simulink model "Lab1bPartC1"  (R2023b)
settings: Solver=VariableStepAuto  StartTime=0.0  StopTime=150  RelTol=1e-3
settings Model: Creator=tanvi  LastModifiedBy=tanvi

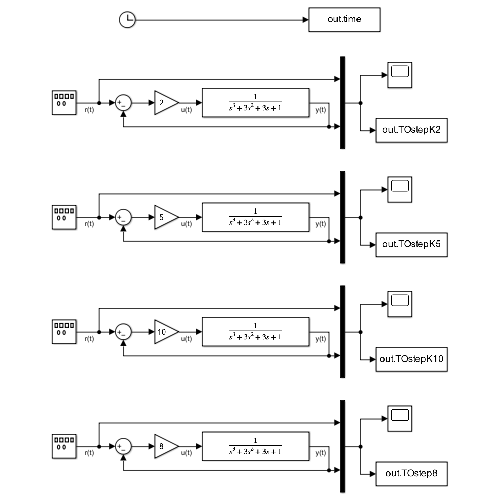
[thumbnail: Simulink's stored preview of the top-level diagram]
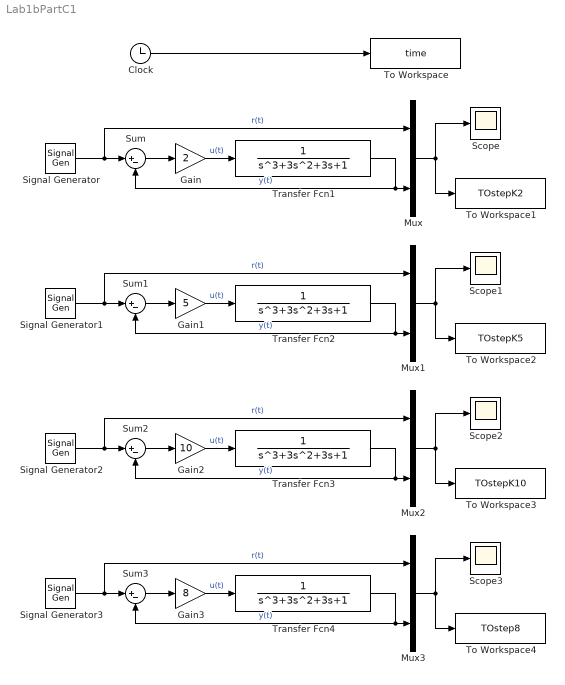
== system Lab1bPartC1 ==
  Clock : Clock
      settings: Decimation=100
  Gain : Gain  Gain=2
  Gain1 : Gain  Gain=5
  Gain2 : Gain  Gain=10
  Gain3 : Gain  Gain=8
  Mux{,1..3} (4 alike) : Mux  Inputs=2
  Scope{,1..3} (4 alike) : Scope
  Signal Generator{,1..3} (4 alike) : SignalGenerator  WaveForm=square  Frequency=0.01
  Sum{,1..3} (4 alike) : Sum  Inputs=|+-
  To Workspace : ToWorkspace  VariableName=time  SampleTime=-1
  To Workspace1 : ToWorkspace  VariableName=TOstepK2  SampleTime=-1
  To Workspace2 : ToWorkspace  VariableName=TOstepK5  SampleTime=-1
  To Workspace3 : ToWorkspace  VariableName=TOstepK10  SampleTime=-1
  To Workspace4 : ToWorkspace  VariableName=TOstep8  SampleTime=-1
  Transfer Fcn{1..4} (4 alike) : TransferFcn  Denominator=[1 3 3 1]
  wires:
  Mux/1 -> Scope/1, To Workspace1/1
  Clock/1 -> To Workspace/1
  Sum/1 -> Gain/1
  Gain/1 -> Transfer Fcn1/1  "u(t)"
  Transfer Fcn1/1 -> Sum/2, Mux/2  "y(t)"
  Signal Generator/1 -> Mux/1, Sum/1  "r(t)"
  Signal Generator1/1 -> Mux1/1, Sum1/1  "r(t)"
  Gain1/1 -> Transfer Fcn2/1  "u(t)"
  Sum1/1 -> Gain1/1
  Mux1/1 -> Scope1/1, To Workspace2/1
  Transfer Fcn2/1 -> Sum1/2, Mux1/2  "y(t)"
  Signal Generator2/1 -> Mux2/1, Sum2/1  "r(t)"
  Gain2/1 -> Transfer Fcn3/1  "u(t)"
  Sum2/1 -> Gain2/1
  Mux2/1 -> Scope2/1, To Workspace3/1
  Transfer Fcn3/1 -> Sum2/2, Mux2/2  "y(t)"
  Mux3/1 -> Scope3/1, To Workspace4/1
  Transfer Fcn4/1 -> Sum3/2, Mux3/2  "y(t)"
  Sum3/1 -> Gain3/1
  Gain3/1 -> Transfer Fcn4/1  "u(t)"
  Signal Generator3/1 -> Mux3/1, Sum3/1  "r(t)"
